simulink model "Practica_1_Simulink"  (R2018a)
settings: Solver=VariableStepAuto  StartTime=0.0  StopTime=100.0  RelTol=1e-3
values from neighbouring files (symbols this model uses):
  a = 0.1    [pactica1.m]
  A = 1    [pactica1.m]
  g = 9.81    [Practica 1.3.m]    (also in pactica1.m = 9.8; practica1Parte2.m)
settings Model: Creator=rafaelbeltranhernandez  LastModifiedBy=rafaelbeltranhernandez

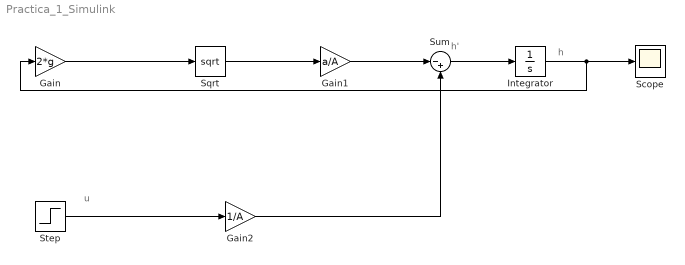
== system Practica_1_Simulink ==
  note: u
  note: h
  note: h'
  Gain : Gain  Gain=2*g
  Gain1 : Gain  Gain=a/A
  Gain2 : Gain  Gain=1/A
  Integrator : Integrator
  Scope : Scope
  Sqrt : Sqrt  SaturateOnIntegerOverflow=on
  Step : Step  After=3  SampleTime=0
  Sum : Sum  Inputs=|-+
  wires:
  Integrator/1 -> Gain/1, Scope/1
  Sum/1 -> Integrator/1
  Gain1/1 -> Sum/1
  Sqrt/1 -> Gain1/1
  Gain/1 -> Sqrt/1
  Step/1 -> Gain2/1
  Gain2/1 -> Sum/2
